simulink model "W6_cs"  (Simulink 8.3)
settings: Solver=ode4  SolverMode=SingleTasking  StartTime=0.0  StopTime=inf  FixedStep=1/60  RelTol=1e-3
model workspace (MAT data in the model file):
  mbox_table : struct (value not decoded)
  model_closed = 0
  sim_status = 0
PreLoadFcn:
  | check_NUTS_defined;
  | 
  | assignin('base',['model_closed_' bdroot],false);
InitFcn:
  | PreScanExperimentInitFcn(bdroot)
StopFcn:
  | PreScanExperimentStopFcn(bdroot)
  | close all;
  | 
  | format shortg
  | c = clock;
  | log_filename = ['log_EXT_',num2str(c(1)),'_',num2str(c(2)),'_',num2str(c(3)),'_',num2str(c(4)),'_',num2str(c(5)),'_',num2str(round(c(6)))];
  | save(log_filename,'res')
undefined symbols (not defined in the file): DiscIntNeverNeededParam, gray, warningInitialVelocity, x0
libraries: simulink x39, PreScanSimulinkLibrary x19, PreScanUsefulBlocks x10, simulink_extras x3, visionsources x2, dspsigops x2, dspnetwork x1, vrlib x1, visionsinks x1
(part 1 of 6)
CloseFcn:
  | evalin('base',['clear model_closed_' bdroot]);
settings Model: Creator=PRESCAN  LastModifiedBy=DrivingSim
settings DataIOCC: LimitDataPoints=off  SaveOutput=off  SignalLogging=off  DSMLogging=off  SaveTime=off
settings OptimizationCC: ExpressionDepthLimit=2147483647  InitFltsAndDblsToZero=on
settings DebuggingCC: SaveWithParameterizedLinksMsg=none  SignalResolutionControl=TryResolveAllWithWarning  SolverPrmCheckMsg=none  MultiTaskDSMMsg=warning  MultiTaskCondExecSysMsg=none  FcnCallInpInsideContextMsg=UseLocalSettings  FrameProcessingCompatibilityMsg=error
settings SFSimCC: SFSimEnableDebug=off  SFSimOverflowDetection=off  SFSimEcho=off
settings GRTTargetCC: TargetFcnLib=ansi_tfl_tmw.mat
settings ConfigComp: CovMetricSettings=dw  CovHtmlReporting=on  CovSaveCumulativeToWorkspaceVar=on  CovSaveSingleToWorkspaceVar=on  CovModelRefEnable=Off  CovExternalEMLEnable=off

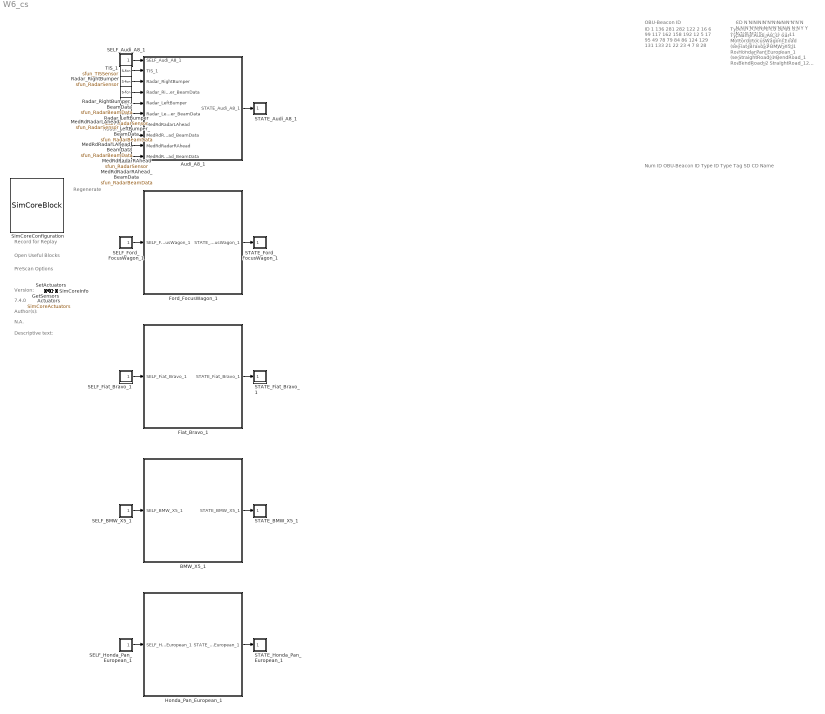
== system W6_cs ==
  note: Regenerate
  note: Record for Replay
  note: Open Useful Blocks
  note: PreScan Options
  note: Version:
  note: 7.4.0
  note: Author(s):
  note: N.A.
  note: Descriptive text:
  note: Num ID OBU-Beacon ID Type ID Type Tag SD CD Name
  note: ID
      |
      | 1
      | 136
      | 281
      | 282
      | 122
      | 2
      | 16
      | 6
      | 99
      | 117
      | 162
      | 158
      | 192
      | 12
      | 5
      | 17
      | 95
      | 49
      | 78
      | 79
      | 84
      | 86
      | 124
      | 129
      | 131
      | 133
      | 21
      | 22
      | 23
      | 4
      | 7
      | 8
      | 28
  note: OBU-Beacon ID
  note: TypeID
      |
      | 1
      | 1
      | 1
      | 1
      | 2
      | 11
      | 11
      | 11
      | 11
      | 11
      | 11
      | 11
      | 11
      | 11
      | 11
      | 11
      | 11
      | 11
      | 11
      | 11
      | 11
      | 11
      | 11
      | 11
      | 11
      | 11
      | 11
      | 11
      | 11
      | 11
      | 11
      | 11
      | 11
  note: TypeTag
      |
      | Car
      | Car
      | Car
      | Car
      | Motor
      | Road (segment)
      | Road (segment)
      | Road (segment)
      | Road (segment)
      | Road (segment)
      | Road (segment)
      | Road (segment)
      | Road (segment)
      | Road (segment)
      | Road (segment)
      | Road (segment)
      | Road (segment)
      | Road (segment)
      | Road (segment)
      | Road (segment)
      | Road (segment)
      | Road (segment)
      | Road (segment)
      | Road (segment)
      | Road (segment)
      | Road (segment)
      | Road (segment)
      | Road (segment)
      | Road (segment)
      | Road (segment)
      | Road (segment)
      | Road (segment)
      | Road (segment)
  note: SD
      |
      | Y
      | Y
      | N
      | N
      | N
      | Y
      | Y
      | Y
      | Y
      | Y
      | Y
      | Y
      | Y
      | Y
      | Y
      | Y
      | Y
      | Y
      | Y
      | Y
      | Y
      | Y
      | Y
      | Y
      | Y
      | Y
      | Y
      | Y
      | Y
      | Y
      | Y
      | Y
      | Y
  note: CD
      |
      | N
      | N
      | N
      | N
      | N
      | N
      | N
      | N
      | N
      | N
      | N
      | N
      | N
      | N
      | N
      | N
      | N
      | N
      | N
      | N
      | N
      | N
      | N
      | N
      | N
      | N
      | N
      | N
      | N
      | N
      | N
      | N
      | N
  note: Name
      |
      | Audi_A8_1
      | Ford_FocusWagon_1
      | Fiat_Bravo_1
      | BMW_X5_1
      | Honda_Pan_European_1
      | StraightRoad_1
      | BendRoad_1
      | BendRoad_2
      | StraightRoad_12
      | StraightRoad_20
      | BendRoad_19
      | BendRoad_17
      | StraightRoad_30
      | BendRoad_3
      | StraightRoad_2
      | BendRoad_4
      | StraightRoad_7
      | Ramp_3
      | Ramp_6
      | Ramp_7
      | Ramp_8
      | StraightRoad_8
      | StraightRoad_14
      | StraightRoad_15
      | BendRoad_11
      | StraightRoad_17
      | StraightRoad_13
      | StraightRoad_16
      | StraightRoad_9
      | StraightRoad_5
      | StraightRoad_3
      | StraightRoad_4
      | StraightRoad_6
  Actuators : DataStoreMemory  Tag=Actuators  DataStoreName=SimCoreActuators  InitialValue=zeros(75,1)
      settings: DeleteFcn=PreScanBlockDeleteFcn;
  Audi_A8_1 : Subsystem  Tag=WorldObjectSubSystem  InitFcn=|
      | UniqueId = '3687';
      | UniqueId = '4148';
      mask Display: image(imread('Audi_A8.jpg'));color('white');text(0,0,' ID=1\n')
  BMW_X5_1 : Subsystem  Tag=WorldObjectSubSystem  InitFcn=UniqueId = '5788';
      mask Display: image(imread('BMW_X5.jpg'));color('white');text(0,0,' ID=282\n')
  Fiat_Bravo_1 : Subsystem  Tag=WorldObjectSubSystem  InitFcn=UniqueId = '4829';
      mask Display: image(imread('Fiat_Bravo.jpg'));color('white');text(0,0,' ID=281\n')
  Ford_FocusWagon_1 : Subsystem  Tag=WorldObjectSubSystem  InitFcn=UniqueId = '4410';
      mask Display: image(imread('Ford_FocusWagon.jpg'));color('white');text(0,0,' ID=136\n')
  GetSensors : Subsystem  Tag=GetSensors  Priority=2  mask(PreScan Simulation Core Block){NrOfSensors=40, TimeStep=1/60}
      mask prompts: NrOfSensors "Number of sensor values"; TimeStep "Timestep [s]"
      mask help:
      | Please do not remove this block from the PreScan compilation sheet,
      | as it contains essential configuration parameters for a PreScan simulation.
      settings: DeleteFcn=PreScanBlockDeleteFcn;
  Honda_Pan_European_1 : Subsystem  Tag=WorldObjectSubSystem  InitFcn=UniqueId = '6490';
      mask Display: image(imread('Honda_Pan_European.jpg'));color('white');text(0,0,' ID=122\n')
  MedRdRadarLAhead : S-Function  Priority=3  LoadFcn=load('PrescanScannerSensorData.mat');load('PrescanScannerSensorMessage.mat')  FunctionName=sfun_RadarSensor  Parameters=timestepMask maxInputMessages maxOutputMessages sensorID detectableObjects  EnableBusSupport=off  mask{timestepMask=1/60, maxInputMessages=0, maxOutputMessages=1, sensorID=6836, detectableObjects=1}
      mask prompts: timestepMask "MATLAB timestep:"; maxInputMessages "Max input messages:"; maxOutputMessages "Max output messages:"; sensorID "Sensor ID:"; detectableObjects "Max detectable objects:"
      mask help: RadarSensor I/O
      mask Display: image(imread('Radar.png'))
  MedRdRadarLAhead_BeamData : S-Function  Priority=3  LoadFcn=load('PrescanScannerSensorBeamData.mat');load('PrescanScannerSensorBeamMessage.mat')  FunctionName=sfun_RadarBeamData  Parameters=timestepMask maxInputMessages maxOutputMessages sensorID detectableObjects  EnableBusSupport=off  mask{timestepMask=1/60, maxInputMessages=0, maxOutputMessages=1, sensorID=6836, detectableObjects=1}
      mask prompts: timestepMask "MATLAB timestep:"; maxInputMessages "Max input messages:"; maxOutputMessages "Max output messages:"; sensorID "Sensor ID:"; detectableObjects "Max detectable objects:"
      mask help: RadarSensor I/O
      mask Display: image(imread('BeamInfo.png'))
  MedRdRadarRAhead : S-Function  Priority=3  LoadFcn=load('PrescanScannerSensorData.mat');load('PrescanScannerSensorMessage.mat')  FunctionName=sfun_RadarSensor  Parameters=timestepMask maxInputMessages maxOutputMessages sensorID detectableObjects  EnableBusSupport=off  mask{timestepMask=1/60, maxInputMessages=0, maxOutputMessages=1, sensorID=6837, detectableObjects=1}
      mask prompts: timestepMask "MATLAB timestep:"; maxInputMessages "Max input messages:"; maxOutputMessages "Max output messages:"; sensorID "Sensor ID:"; detectableObjects "Max detectable objects:"
      mask help: RadarSensor I/O
      mask Display: image(imread('Radar.png'))
  MedRdRadarRAhead_BeamData : S-Function  Priority=3  LoadFcn=load('PrescanScannerSensorBeamData.mat');load('PrescanScannerSensorBeamMessage.mat')  FunctionName=sfun_RadarBeamData  Parameters=timestepMask maxInputMessages maxOutputMessages sensorID detectableObjects  EnableBusSupport=off  mask{timestepMask=1/60, maxInputMessages=0, maxOutputMessages=1, sensorID=6837, detectableObjects=1}
      mask prompts: timestepMask "MATLAB timestep:"; maxInputMessages "Max input messages:"; maxOutputMessages "Max output messages:"; sensorID "Sensor ID:"; detectableObjects "Max detectable objects:"
      mask help: RadarSensor I/O
      mask Display: image(imread('BeamInfo.png'))
  Radar_LeftBumper : S-Function  Priority=3  LoadFcn=load('PrescanScannerSensorData.mat');load('PrescanScannerSensorMessage.mat')  FunctionName=sfun_RadarSensor  Parameters=timestepMask maxInputMessages maxOutputMessages sensorID detectableObjects  EnableBusSupport=off  mask{timestepMask=1/60, maxInputMessages=0, maxOutputMessages=1, sensorID=6637, detectableObjects=1}
      mask prompts: timestepMask "MATLAB timestep:"; maxInputMessages "Max input messages:"; maxOutputMessages "Max output messages:"; sensorID "Sensor ID:"; detectableObjects "Max detectable objects:"
      mask help: RadarSensor I/O
      mask Display: image(imread('Radar.png'))
  Radar_LeftBumper_BeamData : S-Function  Priority=3  LoadFcn=load('PrescanScannerSensorBeamData.mat');load('PrescanScannerSensorBeamMessage.mat')  FunctionName=sfun_RadarBeamData  Parameters=timestepMask maxInputMessages maxOutputMessages sensorID detectableObjects  EnableBusSupport=off  mask{timestepMask=1/60, maxInputMessages=0, maxOutputMessages=1, sensorID=6637, detectableObjects=1}
      mask prompts: timestepMask "MATLAB timestep:"; maxInputMessages "Max input messages:"; maxOutputMessages "Max output messages:"; sensorID "Sensor ID:"; detectableObjects "Max detectable objects:"
      mask help: RadarSensor I/O
      mask Display: image(imread('BeamInfo.png'))
  Radar_RightBumper : S-Function  Priority=3  LoadFcn=load('PrescanScannerSensorData.mat');load('PrescanScannerSensorMessage.mat')  FunctionName=sfun_RadarSensor  Parameters=timestepMask maxInputMessages maxOutputMessages sensorID detectableObjects  EnableBusSupport=off  mask{timestepMask=1/60, maxInputMessages=0, maxOutputMessages=1, sensorID=6636, detectableObjects=1}
      mask prompts: timestepMask "MATLAB timestep:"; maxInputMessages "Max input messages:"; maxOutputMessages "Max output messages:"; sensorID "Sensor ID:"; detectableObjects "Max detectable objects:"
      mask help: RadarSensor I/O
      mask Display: image(imread('Radar.png'))
  Radar_RightBumper_BeamData : S-Function  Priority=3  LoadFcn=load('PrescanScannerSensorBeamData.mat');load('PrescanScannerSensorBeamMessage.mat')  FunctionName=sfun_RadarBeamData  Parameters=timestepMask maxInputMessages maxOutputMessages sensorID detectableObjects  EnableBusSupport=off  mask{timestepMask=1/60, maxInputMessages=0, maxOutputMessages=1, sensorID=6636, detectableObjects=1}
      mask prompts: timestepMask "MATLAB timestep:"; maxInputMessages "Max input messages:"; maxOutputMessages "Max output messages:"; sensorID "Sensor ID:"; detectableObjects "Max detectable objects:"
      mask help: RadarSensor I/O
      mask Display: image(imread('BeamInfo.png'))
  SELF_Audi_A8_1 : Subsystem  Tag=SELF  Priority=3  mask(PreScan Source Block: SELF){PortName=SELF_Audi_A8_1, PortIndex=0, PortWidth=8, TimeStep=1/60}
      mask prompts: PortName "Auto-Assigned: Port Name [-]"; PortIndex "Auto-Assigned: Port Index [-]"; PortWidth "Auto-Assigned: Port Dimensions"; TimeStep "Auto-Assigned: Upload Period [s]"
      mask help:
      | The SELF port shows (state) information of the actor itself. The outputs are position in the experiment's axis system and the GPS coordinates, and the object's absolute velocity and compass heading.
      |
      | For more information, please click Help.
      settings: DeleteFcn=PreScanBlockDeleteFcn;
      mask Help: eval('openHelp(462)')
      mask Display: image(imread('GPS.png'))
  SELF_BMW_X5_1 : Subsystem  Tag=SELF  Priority=3  mask(PreScan Source Block: SELF){PortName=SELF_BMW_X5_1, PortIndex=24, PortWidth=8, TimeStep=1/60}
      mask prompts: PortName "Auto-Assigned: Port Name [-]"; PortIndex "Auto-Assigned: Port Index [-]"; PortWidth "Auto-Assigned: Port Dimensions"; TimeStep "Auto-Assigned: Upload Period [s]"
      mask help:
      | The SELF port shows (state) information of the actor itself. The outputs are position in the experiment's axis system and the GPS coordinates, and the object's absolute velocity and compass heading.
      |
      | For more information, please click Help.
      settings: DeleteFcn=PreScanBlockDeleteFcn;
      mask Help: eval('openHelp(462)')
      mask Display: image(imread('GPS.png'))
  SELF_Fiat_Bravo_1 : Subsystem  Tag=SELF  Priority=3  mask(PreScan Source Block: SELF){PortName=SELF_Fiat_Bravo_1, PortIndex=16, PortWidth=8, TimeStep=1/60}
      mask prompts: PortName "Auto-Assigned: Port Name [-]"; PortIndex "Auto-Assigned: Port Index [-]"; PortWidth "Auto-Assigned: Port Dimensions"; TimeStep "Auto-Assigned: Upload Period [s]"
      mask help:
      | The SELF port shows (state) information of the actor itself. The outputs are position in the experiment's axis system and the GPS coordinates, and the object's absolute velocity and compass heading.
      |
      | For more information, please click Help.
      settings: DeleteFcn=PreScanBlockDeleteFcn;
      mask Help: eval('openHelp(462)')
      mask Display: image(imread('GPS.png'))
  SELF_Ford_FocusWagon_1 : Subsystem  Tag=SELF  Priority=3  mask(PreScan Source Block: SELF){PortName=SELF_Ford_FocusWagon_1, PortIndex=8, PortWidth=8, TimeStep=1/60}
      mask prompts: PortName "Auto-Assigned: Port Name [-]"; PortIndex "Auto-Assigned: Port Index [-]"; PortWidth "Auto-Assigned: Port Dimensions"; TimeStep "Auto-Assigned: Upload Period [s]"
      mask help:
      | The SELF port shows (state) information of the actor itself. The outputs are position in the experiment's axis system and the GPS coordinates, and the object's absolute velocity and compass heading.
      |
      | For more information, please click Help.
      settings: DeleteFcn=PreScanBlockDeleteFcn;
      mask Help: eval('openHelp(462)')
      mask Display: image(imread('GPS.png'))
  SELF_Honda_Pan_European_1 : Subsystem  Tag=SELF  Priority=3  mask(PreScan Source Block: SELF){PortName=SELF_Honda_Pan_European_1, PortIndex=32, PortWidth=8, TimeStep=1/60}
      mask prompts: PortName "Auto-Assigned: Port Name [-]"; PortIndex "Auto-Assigned: Port Index [-]"; PortWidth "Auto-Assigned: Port Dimensions"; TimeStep "Auto-Assigned: Upload Period [s]"
      mask help:
      | The SELF port shows (state) information of the actor itself. The outputs are position in the experiment's axis system and the GPS coordinates, and the object's absolute velocity and compass heading.
      |
      | For more information, please click Help.
      settings: DeleteFcn=PreScanBlockDeleteFcn;
      mask Help: eval('openHelp(462)')
      mask Display: image(imread('GPS.png'))
  STATE_Audi_A8_1 : Subsystem  Tag=State  Priority=0  mask(PreScan Sink Block: State){x0=-399.91707801225488, y0=254.16247682781102, z0=0.55, Roll0=0, Pitch0=0, Yaw0=339.99999999999989, TimeStep=1/60}
      mask prompts: x0 "Ini x-position VEHICLE wrt GLOBAL axis system [m]"; y0 "Ini y-position VEHICLE wrt GLOBAL axis system [m]"; z0 "Ini z-position VEHICLE wrt GLOBAL axis system [m]"; Roll0 "Ini roll-angle BODY wrt VEHICLE axis system [deg]"; Pitch0 "Ini pitch-angle BODY wrt VEHICLE axis system [deg]"; Yaw0 "Ini yaw-angle VEHICLE wrt GLOBAL axis system [deg]"; TimeStep "Time Step [s]"
      mask help:
      | The Actor State contains a vector signal of size (9x1), containing the following signals:
      |
      | -  Position                  (x,y,z)                                     [m]
      | -  Velocity                  (vx,vy,vz)                               [m/s]
      | -  Angles                    (Roll, Pitch, Yaw)                   [rad]
      |
      | The Actor state is defined in the global axis system.
      | The state is superponed on the Initial position defined in the GUI.
      |
      | For more information, please click Help.
      settings: DeleteFcn=PreScanBlockDeleteFcn;
      mask Help: eval('openHelp(222)')
      mask Display: image(imread('State.png'))
  STATE_BMW_X5_1 : Subsystem  Tag=State  Priority=0  mask(PreScan Sink Block: State){x0=-66.9525002880753, y0=135.98733029367131, z0=0.69, Roll0=0, Pitch0=0, Yaw0=160.19495482924066, TimeStep=1/60}
      mask prompts: x0 "Ini x-position VEHICLE wrt GLOBAL axis system [m]"; y0 "Ini y-position VEHICLE wrt GLOBAL axis system [m]"; z0 "Ini z-position VEHICLE wrt GLOBAL axis system [m]"; Roll0 "Ini roll-angle BODY wrt VEHICLE axis system [deg]"; Pitch0 "Ini pitch-angle BODY wrt VEHICLE axis system [deg]"; Yaw0 "Ini yaw-angle VEHICLE wrt GLOBAL axis system [deg]"; TimeStep "Time Step [s]"
      mask help:
      | The Actor State contains a vector signal of size (9x1), containing the following signals:
      |
      | -  Position                  (x,y,z)                                     [m]
      | -  Velocity                  (vx,vy,vz)                               [m/s]
      | -  Angles                    (Roll, Pitch, Yaw)                   [rad]
      |
      | The Actor state is defined in the global axis system.
      | The state is superponed on the Initial position defined in the GUI.
      |
      | For more information, please click Help.
      settings: DeleteFcn=PreScanBlockDeleteFcn;
      mask Help: eval('openHelp(222)')
      mask Display: image(imread('State.png'))
  STATE_Fiat_Bravo_1 : Subsystem  Tag=State  Priority=0  mask(PreScan Sink Block: State){x0=870.78469646749215, y0=-350.59511540043718, z0=0.56, Roll0=0, Pitch0=0, Yaw0=72.606570567857887, TimeStep=1/60}
      mask prompts: x0 "Ini x-position VEHICLE wrt GLOBAL axis system [m]"; y0 "Ini y-position VEHICLE wrt GLOBAL axis system [m]"; z0 "Ini z-position VEHICLE wrt GLOBAL axis system [m]"; Roll0 "Ini roll-angle BODY wrt VEHICLE axis system [deg]"; Pitch0 "Ini pitch-angle BODY wrt VEHICLE axis system [deg]"; Yaw0 "Ini yaw-angle VEHICLE wrt GLOBAL axis system [deg]"; TimeStep "Time Step [s]"
      mask help:
      | The Actor State contains a vector signal of size (9x1), containing the following signals:
      |
      | -  Position                  (x,y,z)                                     [m]
      | -  Velocity                  (vx,vy,vz)                               [m/s]
      | -  Angles                    (Roll, Pitch, Yaw)                   [rad]
      |
      | The Actor state is defined in the global axis system.
      | The state is superponed on the Initial position defined in the GUI.
      |
      | For more information, please click Help.
      settings: DeleteFcn=PreScanBlockDeleteFcn;
      mask Help: eval('openHelp(222)')
      mask Display: image(imread('State.png'))
  STATE_Ford_FocusWagon_1 : Subsystem  Tag=State  Priority=0  mask(PreScan Sink Block: State){x0=-113.09931945800781, y0=149.31063842773437, z0=0.5, Roll0=0, Pitch0=0, Yaw0=340.09422131164354, TimeStep=1/60}
      mask prompts: x0 "Ini x-position VEHICLE wrt GLOBAL axis system [m]"; y0 "Ini y-position VEHICLE wrt GLOBAL axis system [m]"; z0 "Ini z-position VEHICLE wrt GLOBAL axis system [m]"; Roll0 "Ini roll-angle BODY wrt VEHICLE axis system [deg]"; Pitch0 "Ini pitch-angle BODY wrt VEHICLE axis system [deg]"; Yaw0 "Ini yaw-angle VEHICLE wrt GLOBAL axis system [deg]"; TimeStep "Time Step [s]"
      mask help:
      | The Actor State contains a vector signal of size (9x1), containing the following signals:
      |
      | -  Position                  (x,y,z)                                     [m]
      | -  Velocity                  (vx,vy,vz)                               [m/s]
      | -  Angles                    (Roll, Pitch, Yaw)                   [rad]
      |
      | The Actor state is defined in the global axis system.
      | The state is superponed on the Initial position defined in the GUI.
      |
      | For more information, please click Help.
      settings: DeleteFcn=PreScanBlockDeleteFcn;
      mask Help: eval('openHelp(222)')
      mask Display: image(imread('State.png'))
  STATE_Honda_Pan_European_1 : Subsystem  Tag=State  Priority=0  mask(PreScan Sink Block: State){x0=1149.497802734375, y0=222.82337188720703, z0=0.5949, Roll0=0, Pitch0=0, Yaw0=170, TimeStep=1/60}
      mask prompts: x0 "Ini x-position VEHICLE wrt GLOBAL axis system [m]"; y0 "Ini y-position VEHICLE wrt GLOBAL axis system [m]"; z0 "Ini z-position VEHICLE wrt GLOBAL axis system [m]"; Roll0 "Ini roll-angle BODY wrt VEHICLE axis system [deg]"; Pitch0 "Ini pitch-angle BODY wrt VEHICLE axis system [deg]"; Yaw0 "Ini yaw-angle VEHICLE wrt GLOBAL axis system [deg]"; TimeStep "Time Step [s]"
      mask help:
      | The Actor State contains a vector signal of size (9x1), containing the following signals:
      |
      | -  Position                  (x,y,z)                                     [m]
      | -  Velocity                  (vx,vy,vz)                               [m/s]
      | -  Angles                    (Roll, Pitch, Yaw)                   [rad]
      |
      | The Actor state is defined in the global axis system.
      | The state is superponed on the Initial position defined in the GUI.
      |
      | For more information, please click Help.
      settings: DeleteFcn=PreScanBlockDeleteFcn;
      mask Help: eval('openHelp(222)')
      mask Display: image(imread('State.png'))
  SetActuators : Subsystem  Tag=SetActuators  Priority=1  mask(PreScan Simulation Core Block){TimeStep=1/60, NrOfActuators=75}
      mask prompts: TimeStep "Timestep [s]"; NrOfActuators "Number of actuator values"
      mask help:
      | Please do not remove this block from the PreScan compilation sheet,
      | as it contains essential configuration parameters for a PreScan simulation.
      settings: DeleteFcn=PreScanBlockDeleteFcn;
  SimCoreConfiguration : M-S-Function  Tag=SimCoreConfiguration  Description=2DB88F1AB85D6AB0C7A46FBF0985E444AD6743D233D065952F88CD829B0DCDCE  FunctionName=SimCoreBlock  Parameters=ExperimentXML PortsXML SimulationCore HostName CheckStart EnableLog RfR EnableGPUAccel ShowComputationTime  mask(PreScan Simulation Core Configurator){SimulationCore=NUTS, HostName=0, CheckStart=0, prescanversion='7.4.0', EnableLog=off, RfR=0, EnableGPUAccel=on, ShowComputationTime=off}
      mask prompts: SimulationCore "Simulation Core"; HostName "Simulation Host"; CheckStart "Show START Dialog"; prescanversion "PreScan Version"; EnableLog "Create TA Log"; RfR "Record for Replay"; EnableGPUAccel "Enable GPU Acceleration"; ShowComputationTime "Show ComputationTime Scope"
      mask help:
      | Please do not remove this block from the PreScan compilation sheet,
      | as it contains essential configuration parameter for a PreScan simulation.
      mask init:
      | model = bdroot;
      | ExperimentXML = [model(1:end-3) '.pex'];
      | PortsXML = [model '_ports.pcd'];
      settings: DeleteFcn=PreScanBlockDeleteFcn;  ModelCloseFcn=assignin('base',['model_closed_' bdroot],true);
      mask Help: eval('openHelp(812)')
      mask Display: image(imread('prescanlogo.ico'))
  SimCoreInfo : Subsystem  Tag=SimCoreInfo
  TIS_1 : S-Function  Priority=3  LoadFcn=load('PrescanScannerSensorData.mat');load('PrescanScannerSensorMessage.mat')  FunctionName=sfun_TISSensor  Parameters=timestepMask maxInputMessages maxOutputMessages sensorID detectableObjects  EnableBusSupport=off  mask{timestepMask=1/60, maxInputMessages=0, maxOutputMessages=1, sensorID=4973, detectableObjects=1}
      mask prompts: timestepMask "MATLAB timestep:"; maxInputMessages "Max input messages:"; maxOutputMessages "Max output messages:"; sensorID "Sensor ID:"; detectableObjects "Max detectable objects:"
      mask help: TIS Sensor I/O
      mask Display: image(imread('TIS.png'))
  wires:
  SetActuators/1(dummy) -> GetSensors/1(dummy)
  Audi_A8_1/1(STATE_Audi_A8_1) -> STATE_Audi_A8_1/1(State)
  SELF_Audi_A8_1/1(U) -> Audi_A8_1/1(SELF_Audi_A8_1)
  TIS_1/1 -> Audi_A8_1/2(TIS_1)
  Radar_RightBumper/1 -> Audi_A8_1/3(Radar_RightBumper)
  Radar_RightBumper_BeamData/1 -> Audi_A8_1/4(Radar_RightBumper_BeamData)
  Radar_LeftBumper/1 -> Audi_A8_1/5(Radar_LeftBumper)
  Radar_LeftBumper_BeamData/1 -> Audi_A8_1/6(Radar_LeftBumper_BeamData)
  MedRdRadarLAhead/1 -> Audi_A8_1/7(MedRdRadarLAhead)
  MedRdRadarLAhead_BeamData/1 -> Audi_A8_1/8(MedRdRadarLAhead_BeamData)
  MedRdRadarRAhead/1 -> Audi_A8_1/9(MedRdRadarRAhead)
  MedRdRadarRAhead_BeamData/1 -> Audi_A8_1/10(MedRdRadarRAhead_BeamData)
  Ford_FocusWagon_1/1(STATE_Ford_FocusWagon_1) -> STATE_Ford_FocusWagon_1/1(State)
  SELF_Ford_FocusWagon_1/1(U) -> Ford_FocusWagon_1/1(SELF_Ford_FocusWagon_1)
  Fiat_Bravo_1/1(STATE_Fiat_Bravo_1) -> STATE_Fiat_Bravo_1/1(State)
  SELF_Fiat_Bravo_1/1(U) -> Fiat_Bravo_1/1(SELF_Fiat_Bravo_1)
  BMW_X5_1/1(STATE_BMW_X5_1) -> STATE_BMW_X5_1/1(State)
  SELF_BMW_X5_1/1(U) -> BMW_X5_1/1(SELF_BMW_X5_1)
  Honda_Pan_European_1/1(STATE_Honda_Pan_European_1) -> STATE_Honda_Pan_European_1/1(State)
  SELF_Honda_Pan_European_1/1(U) -> Honda_Pan_European_1/1(SELF_Honda_Pan_European_1)

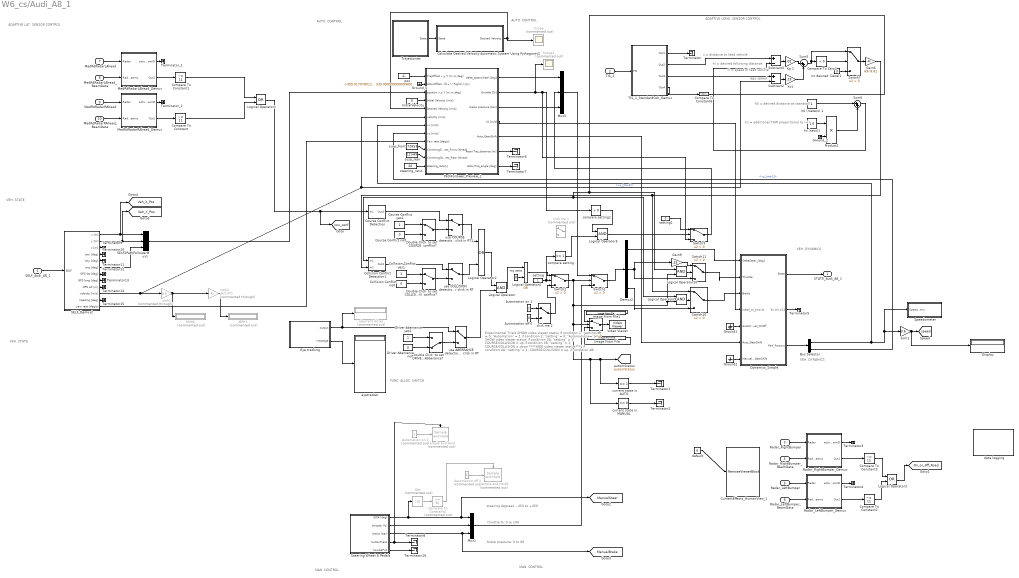
== system W6_cs/Audi_A8_1 ==
  note: Experimental Trials
      | SHOW video viewer status
      | if condition 1; ''setting'' = 0; ''Automation'' = 1
      | if condition 2; ''setting'' = 0; ''Automation'' = 1
      |
      | SHOW video viewer status
      | if condition 3A; ''setting'' = 1; COURSE/COLLISION = up
      | if condition 3B; ''setting'' = 1; COURSE/COLLISION = down
      |
      | ****HIDE video viewer status****
      | if condition 4A; ''setting'' = 1; COURSE/COLLISION = up,
      | if condition 4B; ''setting'' = 1; COURSE/COLLISION = down
      | if condition 4C; "setting"= 0; "Automation" = 0
  note: hi = desired following distance
  note: x = distance to lead vehicle
  note: vi = speed of lead vehicle
  note: hv = additional THW proportional to (vi)
  note: h0 = desired distance at standstill
  note: VEH. STATE
  note: VEH. STATE
  note: AUTO. CONTROL
  note: AUTO. CONTROL
  note: VEH. DYNAMICS
  note: VEH. DYNAMICS
  note: FUNC. ALLOC. SWITCH
  note: throttle %: 0 to 100
  note: brake pressure: 0 to 69
  note: steering degrees: - 450 to +450
  note: MAN. CONTROL
  note: MAN. CONTROL
  note: ADAPTIVE LONG. SENSOR CONTROL
  note: ADAPTIVE LAT. SENSOR CONTROL
  note: ego speed
  SELF_Audi_A8_1 : Inport  Tag=SELFInport
  TIS_1 : Inport  Tag=RadarInport  Port=2  OutDataTypeStr=Bus: PRESCAN_SCANNERSENSORMESSAGE
  Radar_RightBumper : Inport  Tag=RadarInport  Port=3  OutDataTypeStr=Bus: PRESCAN_SCANNERSENSORMESSAGE
  Radar_RightBumper_BeamData : Inport  Tag=RadarInport  Port=4  OutDataTypeStr=Bus: PRESCAN_SCANNERSENSORBEAMMESSAGE
  Radar_LeftBumper : Inport  Tag=RadarInport  Port=5  OutDataTypeStr=Bus: PRESCAN_SCANNERSENSORMESSAGE
  Radar_LeftBumper_BeamData : Inport  Tag=RadarInport  Port=6  OutDataTypeStr=Bus: PRESCAN_SCANNERSENSORBEAMMESSAGE
  MedRdRadarLAhead : Inport  Tag=RadarInport  Port=7  OutDataTypeStr=Bus: PRESCAN_SCANNERSENSORMESSAGE
  MedRdRadarLAhead_BeamData : Inport  Tag=RadarInport  Port=8  OutDataTypeStr=Bus: PRESCAN_SCANNERSENSORBEAMMESSAGE
  MedRdRadarRAhead : Inport  Tag=RadarInport  Port=9  OutDataTypeStr=Bus: PRESCAN_SCANNERSENSORMESSAGE
  MedRdRadarRAhead_BeamData : Inport  Tag=RadarInport  Port=10  OutDataTypeStr=Bus: PRESCAN_SCANNERSENSORBEAMMESSAGE
  Abs : Abs  Commented=on
  Autiomation off 0 : Constant  Value=0
  Automation off 3 : Constant  Commented=on  Value=0
  Automation on 1 : Constant
  Automation on 2 : Constant  Commented=on
  Bus Selector : BusSelector  OutputSignals=vx_[ms-1],vy_[ms-1]
  Calculate Desired Velocity Automatic System Using Pythagoras2 : Subsystem
  Collision Conflict Detection1 : Subsystem
  Collision Conflict no0 : Constant  Value=0
  Collision Conflict yes1 : Constant
  Compare To Constant{,1..3} (4 alike) : simulink/Logic and Bit Operations/Compare To Constant  relop=~=  const=11  OutDataTypeStr=boolean
  Compare To Constant4 : simulink/Logic and Bit Operations/Compare To Constant  Commented=on  relop=>=  const=90  OutDataTypeStr=boolean
  Compare To Constant6 : simulink/Logic and Bit Operations/Compare To Constant  relop===  const=1  OutDataTypeStr=boolean
  Compare To Zero1 : simulink/Logic and Bit Operations/Compare To Zero  relop=<  OutDataTypeStr=boolean
  Course Conflict Detection : Subsystem
  Course Conflict no0 : Constant  Value=0
  Course Conflict yes1 : Constant
  CurrentEffects_HumanView_1 : M-S-Function  FunctionName=RemoteViewerBlock  Parameters=2
  Demux2 : Demux  Outputs=3
  Display : Display
  Double Click  to set COLLISION  conflict? : ManualSwitch
  Double Click  to set COURSE  conflict? : ManualSwitch
  Double Click  to set DRIVER  Abberance? : ManualSwitch  CurrentSetting=0
  Driver Aberrance no0 : Constant  Value=0
  Driver Aberrance yes1 : Constant
  Dynamics_Simple : Subsystem  Tag=Simple_Vehicle_Dynamics  mask(PreScan Block: Simple Dynamics){Migrate=on, TimeStep=1/60, ComputationMode=Continuous_Time}
      mask prompts: Migrate "Migrate. During migration this block will be replaced by a newer one."; TimeStep "Auto assigned: Time Step [s]"; ComputationMode "Computation mode:"
      mask help:
      | The Simple Dynamics Model is selected in the GUI to simulate vehicle dynamics behavior.
      |
      | The Simple Dynamics Model is completely open to the user. The parameters of this model can be set in the Simple Dynamics dialog in the GUI.
      |
      | For more information, please click Help.
      mask init:
      | p = SimpleDyn_pars;
      settings: DeleteFcn=PreScanBlockDeleteFcn;
      mask Help: eval('openHelp(220)')
      mask Display:
      | image(imread('SimpleDyn.png'))
      | port_label('input', 1, '{\delta}_S_t_ _e_e_r [deg]','texmode','on')
      | port_label('input', 2, 'Throttle [%]')
      | port_label('input', 3, 'Brake Pres [bar]')
      | port_label('input', 4, 'V_0 [ms-1]','texmode','on')
      | port_label('input', 5, 'Auto=[0]/Manual=[1]')
      | port_label('input', 6, 'Auto_GearShift')
      | port_label('input', 7, 'Manual_GearShift')
      | port_label('output', 1, 'State')
      | port_label('output', 2, 'Vx [ms-1]')
      | port_label('output', 3, 'Perf Params')
  Eye tracking : Subsystem
  Gain6 : Gain  Gain=69/-9.81
  Gain9 : Gain  Gain=.25
  Ground1 : Ground
  Ground2 : Ground
  Ground_1 : Ground
  Ground_2 : Ground
  Image From File : visionsources/Image From File  Tag=vipblks_nd  FileName=NormalDrivingGreen.png  imagePorts=One multidimensional signal  Ts=inf  ImageDataType=Inherit from input image  Signed=on  WordLength=16  sdImageDataType=uint(8)  FractionLengthMode=User-defined  FractionLength=15  OutPortLabels=R|G|B
  Image From File1 : visionsources/Image From File  Tag=vipblks_nd  FileName=AutoBackupControlRed.png  imagePorts=One multidimensional signal  Ts=inf  ImageDataType=Inherit from input image  Signed=on  WordLength=16  sdImageDataType=uint(8)  FractionLengthMode=User-defined  FractionLength=15  OutPortLabels=R|G|B
  InitialVelocity : Constant  Tag=InitialVelocity  Value=0
  KMH1 : Display  Commented=on
  Kp 1 : Gain  Gain=.02
  Kv1 : Gain  Gain=.23
  Logical Operator{,5,9..10} (4 alike) : Logic  AllPortsSameDT=off  OutDataTypeStr=boolean
  Logical Operator{1..4} (4 alike) : Logic  Operator=OR  AllPortsSameDT=off  OutDataTypeStr=boolean
  MPH1 : Display  Commented=on
  MedRdRadarLAhead_Demux : Subsystem  TreatAsAtomicUnit=on  mask(PreScan Demux Block: Radar){MAXMESSAGES=1}
      mask prompts: MAXMESSAGES "Number of Objects"
      mask help:
      | The Radar Sensor is a detailed sensor based on a physical radar
      | model that includes Antenna GAIN Maps (AGM) and atmospheric
      | attenuation.
      |
      | For more information, please click Help.
      mask Help: eval('openHelp(431)')
      mask Display:
      | port_label('input',1,'Radar')
      | port_label('output',1,'Radar Data')
  MedRdRadarRAhead_Demux : Subsystem  TreatAsAtomicUnit=on  mask(PreScan Demux Block: Radar){MAXMESSAGES=1}
      mask prompts: MAXMESSAGES "Number of Objects"
      mask help:
      | The Radar Sensor is a detailed sensor based on a physical radar
      | model that includes Antenna GAIN Maps (AGM) and atmospheric
      | attenuation.
      |
      | For more information, please click Help.
      mask Help: eval('openHelp(431)')
      mask Display:
      | port_label('input',1,'Radar')
      | port_label('output',1,'Radar Data')
  Mux1 : Mux  Inputs=3
  Mux3 : Mux  Inputs=3
  PathFollower_Preview_1 : Subsystem  Tag=PathFollower_Preview  mask(PreScan Block: Path Follower with Preview){Migrate=on, FileName='Trajectory_1.mat', mass=1820, Jzz=3746, length_a=2.94 - 1.77, length_l=2.94, Angle_Max_SteeringWheel=500, PreviewTime=1, DelayTime=0.1, LowSpeedLimit=20, MaxSteeringRate=1200, CSSampleTime=1/60, PFIntegrationFrequency=60}
      mask prompts: Migrate "Migrate. During migration this block will be replaced by a newer one."; FileName "Trajectory Name"; mass "Mass vehicle total [kg]"; Jzz "Inertia vehicle around yaw axis [kg m2]"; length_a "Distance between COG and front axle [m]"; length_l "Length of wheelbase [m]"; Angle_Max_SteeringWheel "Maximum steering wheel angle [deg]"; PreviewTime "Preview time [s]"; DelayTime "Delay time [s]"; LowSpeedLimit "Low-speed limit [km/h]"; MaxSteeringRate "Maximum steering wheel angle rate [deg/s]"; CSSampleTime "Compilation Sheet sample time [s]"; PFIntegrationFrequency "Lateral controller frequency [Hz]"
      mask help:
      | The Path Follower Model is selected in the GUI to simulate driver behavior.
      |
      | For more information, please click Help.
      mask init:
      | load(['trajectories/',eval(FileName)])
      | traject=trajectory';
      | 
      | Traj_x=traject(:,2);
      | Traj_y=traject(:,3);
      | Traj_t=traject(2,1);
      | Traj_v=sqrt(traject(:,8).^2+traject(:,9).^2+traject(:,10).^2);
      | 
      | RefreshCounter = (1/CSSampleTime) / (PFIntegrationFrequency); %Compilation sheet frequency/path follower frequency
      | 
      | blockPath = gcb;
      | 
      | clear traject;
      mask Help: eval('openHelp(233)')
  Product1 : Product
  Radar_LeftBumper_Demux : Subsystem  TreatAsAtomicUnit=on  mask(PreScan Demux Block: Radar){MAXMESSAGES=1}
      mask prompts: MAXMESSAGES "Number of Objects"
      mask help:
      | The Radar Sensor is a detailed sensor based on a physical radar
      | model that includes Antenna GAIN Maps (AGM) and atmospheric
      | attenuation.
      |
      | For more information, please click Help.
      mask Help: eval('openHelp(431)')
      mask Display:
      | port_label('input',1,'Radar')
      | port_label('output',1,'Radar Data')
  Radar_RightBumper_Demux : Subsystem  TreatAsAtomicUnit=on  mask(PreScan Demux Block: Radar){MAXMESSAGES=1}
      mask prompts: MAXMESSAGES "Number of Objects"
      mask help:
      | The Radar Sensor is a detailed sensor based on a physical radar
      | model that includes Antenna GAIN Maps (AGM) and atmospheric
      | attenuation.
      |
      | For more information, please click Help.
      mask Help: eval('openHelp(431)')
      mask Display:
      | port_label('input',1,'Radar')
      | port_label('output',1,'Radar Data')
  SELF2PathFollowerMux1 : Mux  Inputs=3
  SELF_Demux2 : Subsystem  Tag=DemuxSELF  mask(PreScan Demux Block:){}
      settings: DeleteFcn=PreScanBlockDeleteFcn;
      mask Display:
      | port_label('output',1,'x [m]')
      | port_label('output',2,'y [m]')
      | port_label('output',3,'z [m]','texmode','on')
      | port_label('output',4,'Rotx [deg]','texmode','on')
      | port_label('output',5,'Roty [deg]','texmode','on')
      | port_label('output',6,'Rotz [deg]','texmode','on')
      | port_label('output',7,'GPS lat [deg]','texmode','on')
      | port_label('output',8,'GPS long [deg]','texmode','on')
      | port_label('output',9,'GPS alt [m]','texmode','on')
      | port_label('output',10,'Velocity [m/s]')
      | port_label('output',11,'Heading [deg]')
      | port_label('output',12,'Yaw rate [deg/s]')
  Sample and Hold : dspsigops/Sample and Hold  Commented=on  trig=Rising edge  initCond=0  latchinput=off
  Sample and Hold1 : dspsigops/Sample and Hold  Commented=on  trig=Rising edge  initCond=1  latchinput=off
  Scope : Scope  Commented=on
      settings: YMin=0  YMax=20
  Scope1 : Scope  Commented=on
      settings: YMin=0  YMax=20
  Speedometer : Subsystem
      mask init:
      | FigHandle = figure(101);
      | set(FigHandle, 'Position', [2150, -275, 400, 400]);
      | set(gcf,'Color','None');
      | ha = axes('units','normalized', 'position',[0,0,1,1]);
      | bg = imread('2016_Audi.jpg');
      | imagesc(bg);
      | set(ha,'handlevisibility','off', ...
      |     'visible','off')
      | uistack(ha,'top');
  Steering Wheel & Pedals : Subsystem
  Subtract2 : Sum  Inputs=+-
  Subtract3 : Sum  Inputs=+-
  Sum5 : Sum  Inputs=|++
  Sum6 : Sum  Inputs=|++
  Switch{,1..3,7,10..11} (7 alike) : Switch  Criteria=u2 > Threshold
  TIS_1_StandardCoh_Demux : Subsystem  TreatAsAtomicUnit=on  mask(PreScan Demux Block: TIS){MAXMESSAGES=1}
      mask prompts: MAXMESSAGES "Number of Objects"
      mask Help: eval('openHelp(441)')
      mask Display:
      | port_label('input',1,'TIS')
      | port_label('output',1,'Beam ID [-]')
      | port_label('output',2,'Range [m]')
      | port_label('output',3,'DopplerVelocity [m/s]')
      | port_label('output',4,'{\theta} [deg]','texmode','on')
      | port_label('output',5,'{\phi} [deg]','texmode','on')
      | port_label('output',6,'Target ID [-]','texmode','on')
      | port_label('output',7,'TIS Data','texmode','on')
  Terminator{,1..16} (17 alike) : Terminator
  Terminator_1 : Terminator
  Terminator_2 : Terminator
  Trajectories : Subsystem  Tag=Trajectories  mask(PreScan Source Block: Trajectories){}
      mask help:
      | The Trajectory block contains the trajectories defined in the PreScan Experiment Editor. The output of the trajectory block is the (vehicle) State.
      |
      | For more information, please click Help.
      settings: DeleteFcn=PreScanBlockDeleteFcn;
      mask Help: eval('openHelp(312)')
      mask Display: image(imread('Trajectory.png'));
  Video Viewer : visionsinks/Video Viewer  inputType=Obsolete7b  imagePorts=One multidimensional signal  useColorMap=off  colormapValue=gray(256)  specRange=off  minInputVal=0  maxInputVal=255  FigPos=[436 537 409 53]  AxisZoom=on  trueSizedOnce=off  OpenAtMdlStart=on  DefaultConfigurationName=vipscopes.VideoViewerScopeCfg
  aberrant driver : Display  Commented=on
  click me 1 : ManualSwitch  Commented=on
  click me 2 : ManualSwitch
  compare setting : simulink/Logic and Bit Operations/Compare To Constant  relop===  const=1  OutDataTypeStr=boolean
  compare setting1 : simulink/Logic and Bit Operations/Compare To Constant  relop=>  const=0  OutDataTypeStr=boolean
  current state is AUTO : simulink/Logic and Bit Operations/Compare To Constant  relop===  const=1  OutDataTypeStr=boolean
  current state is MANUAL : simulink/Logic and Bit Operations/Compare To Constant  relop===  const=0  OutDataTypeStr=boolean
  data logging : Subsystem
  default : Constant  Value=0
  eyetracker : Display
  h0 (meters) 1 : Constant
  hv (secs)1 : Constant  Value=1.6
  kmh1 : Gain  Gain=3.6
  kmh2 : Gain  Commented=through  Gain=3.6
  mph2 : Gain  Commented=through  Gain=.621371
  "my zero " : Constant  Value=0
  no desired  Decel1 : Constant  Value=0
  pos : Constant  Tag=pos  Value=[-399.91707801225488 254.16247682781102 339.99999999999989]
  setting : Constant
  setting1 : Constant  Value=0
  steering_ratio : Constant  Tag=steering_ratio  Value=20
  susp_front : Constant  Tag=susp_front  Value=72653
  susp_rear : Constant  Tag=susp_rear  Value=121449
  use ABERRANCE detection or  click in RT : ManualSwitch
  use COLLISION  detection or click in RT : ManualSwitch
  use COURSE  detection or click in RT1 : ManualSwitch
  STATE_Audi_A8_1 : Outport  Tag=StateOutport
  tag scope: ManualBrake=global, ManualSteer=global, On_or_Off_Road=global, Veh_X_Pos=global, Veh_Y_Pos=global, automStatus=global, cou_conf=global, speed=global
  wires:
  SELF_Demux2/10(velocity [m/s]) -> kmh2/1, Subtract2/2, PathFollower_Preview_1/6(velocity [m/s])
  kmh2/1 -> mph2/1, KMH1/1
  mph2/1 -> MPH1/1
  SELF_Demux2/1(x [m]) -> [Veh_X_Pos], SELF2PathFollowerMux1/1
  SELF_Demux2/2(y [m]) -> [Veh_Y_Pos], SELF2PathFollowerMux1/2
  SELF_Demux2/6(rotz [deg]) -> SELF2PathFollowerMux1/3
  Automation on 1/1 -> click me 2/1
  Autiomation off 0/1 -> click me 2/2
  Dynamics_Simple/2(Vx [m s-1]) -> Terminator5/1
  Switch1/1 -> Demux2/1
  Mux3/1 -> Switch1/1
  Course Conflict yes1/1 -> Double Click  to set COURSE  conflict?/1
  Course Conflict no0/1 -> Double Click  to set COURSE  conflict?/2
  Collision Conflict yes1/1 -> Double Click  to set COLLISION  conflict?/1
  Collision Conflict no0/1 -> Double Click  to set COLLISION  conflict?/2
  Double Click  to set COURSE  conflict?/1 -> use COURSE  detection or click in RT1/2
  Double Click  to set COLLISION  conflict?/1 -> use COLLISION  detection or click in RT/2
  TIS_1_StandardCoh_Demux/2(Out2) -> Subtract3/1
  Subtract2/1 -> Kv1/1
  Kp 1/1 -> Sum5/1
  Kv1/1 -> Sum5/2
  Subtract3/1 -> Kp 1/1
  hv (secs)1/1 -> Product1/1
  Product1/1 -> Sum6/2
  h0 (meters) 1/1 -> Sum6/1
  Sum6/1 -> Subtract3/2
  Compare To Zero1/1 -> Switch7/2
  no desired  Decel1/1 -> Switch7/3
  Switch7/1 -> Gain6/1
  Switch10/1 -> Dynamics_Simple/3(Brake)
  Compare To Constant6/1 -> Logical Operator9/1, Collision Conflict Detection1/1(In1), Logical Operator10/1
  Sum5/1 -> Compare To Zero1/1, Switch7/1
  Gain6/1 -> Switch10/1, Collision Conflict Detection1/2(In2)
  Switch11/1 -> Dynamics_Simple/2(Throttle)
  Gain9/1 -> Switch11/1
  Logical Operator9/1 -> Switch10/2
  Logical Operator10/1 -> Switch11/2
  Ground1/1 -> Dynamics_Simple/5(AutoManual_OnOff)
  Double Click  to set DRIVER  Abberance?/1 -> use ABERRANCE detection or  click in RT/2
  Collision Conflict Detection1/1(Out3) -> use COLLISION  detection or click in RT/1
  SELF_Demux2/7(GPS lat [deg]) -> Terminator12/1
  SELF_Demux2/8(GPS long [deg]) -> Terminator13/1
  SELF_Demux2/9(GPS alt [m]) -> Terminator14/1
  Image From File/1 -> Switch/3
  Image From File1/1 -> Switch/1
  Switch/1 -> Video Viewer/1
  SELF_Audi_A8_1/1 -> SELF_Demux2/1(SELF)
  Compare To Constant/1 -> Logical Operator1/2
  Compare To Constant1/1 -> Logical Operator1/1
  Demux2/2 -> Switch11/3, Gain9/1
  Demux2/3 -> Switch10/3
  Driver Aberrance yes1/1 -> Double Click  to set DRIVER  Abberance?/1
  Driver Aberrance no0/1 -> Double Click  to set DRIVER  Abberance?/2
  Switch2/1 -> Logical Operator10/2, Logical Operator9/2, current state is AUTO/1, [automStatus], current state is MANUAL/1, Switch/2, Switch1/2
  Logical Operator/1 -> Logical Operator4/1
  use ABERRANCE detection or  click in RT/1 -> Logical Operator/2
  use COLLISION  detection or click in RT/1 -> Logical Operator2/2
  Logical Operator2/1 -> Logical Operator/1
  Logical Operator1/1 -> [cou_conf], Course Conflict Detection/1(In1)
  Course Conflict Detection/1(Out3) -> use COURSE  detection or click in RT1/1
  use COURSE  detection or click in RT1/1 -> Logical Operator2/1
  Demux2/1 -> Dynamics_Simple/1(DeltaSteer_[deg])
  SELF_Demux2/12(yaw rate [deg/s]) -> PathFollower_Preview_1/9(Yaw rate [deg/s])
  Dynamics_Simple/3(Perf_Params) -> Bus Selector/1
  PathFollower_Preview_1/4(v0 [m/s]) -> Dynamics_Simple/4(Initial_Vx_[ms-1])
  PathFollower_Preview_1/5(Auto_GearShift) -> Dynamics_Simple/6(Auto_GearShift)
  PathFollower_Preview_1/1(delta_steerwheel [deg]) -> Mux3/1
  PathFollower_Preview_1/3(brake pressure [bar]) -> Mux3/3
  SELF2PathFollowerMux1/1 -> PathFollower_Preview_1/3(position x,y,Y [m,m,deg])
  pos/1 -> PathFollower_Preview_1/1(TrajOffset x,y,Y [m,m,deg])
  InitialVelocity/1 -> PathFollower_Preview_1/4(Initial Velocity [m/s])
  susp_front/1 -> PathFollower_Preview_1/10(CorneringStiffness_Tyres_Front [N/rad])
  susp_rear/1 -> PathFollower_Preview_1/11(CorneringStiffness_Tyres_Rear [N/rad])
  steering_ratio/1 -> PathFollower_Preview_1/12(steering_ratio[-])
  TIS_1/1 -> TIS_1_StandardCoh_Demux/1(TIS)
  Dynamics_Simple/1(State) -> STATE_Audi_A8_1/1
  Ground2/1 -> Dynamics_Simple/7(Manual_GearShift)
  SELF_Demux2/3(z [m]) -> Terminator9/1
  SELF_Demux2/4(rotx [deg]) -> Terminator10/1
  SELF_Demux2/5(roty [deg]) -> Terminator11/1
  SELF_Demux2/11(heading [deg]) -> Terminator15/1
  Bus Selector/1 -> PathFollower_Preview_1/7(vx [m/s]), kmh1/1, Speedometer/1("Speed, m/s")  "<vx_[ms-1]>"
  Bus Selector/2 -> PathFollower_Preview_1/8(vy [m/s])  "<vy_[ms-1]>"
  Mux1/1 -> Switch1/3
  PathFollower_Preview_1/6(Actor/Traj_distance [m]) -> Terminator6/1
  PathFollower_Preview_1/7(Actor/Traj_angle [deg]) -> Terminator7/1
  Eye tracking/1(output) -> use ABERRANCE detection or  click in RT/1, aberrant driver/1
  PathFollower_Preview_1/2(throttle [%]) -> Scope1/1, Switch3/3, compare setting1/1
  Steering Wheel & Pedals/1(SWA (deg)) -> Abs/1, [ManualSteer], Mux1/1
  Steering Wheel & Pedals/2(throttle (%)) -> Mux1/2
  Steering Wheel & Pedals/3(brake (bar)) -> Mux1/3, [ManualBrake]
  Eye tracking/2(message) -> eyetracker/1
  Compare To Constant2/1 -> Logical Operator3/2
  Compare To Constant3/1 -> Logical Operator3/1
  Radar_LeftBumper_Demux/2(Out1) -> Compare To Constant2/1
  Radar_RightBumper_Demux/2(Out1) -> Compare To Constant3/1
  Logical Operator3/1 -> [On_or_Off_Road]
  Radar_LeftBumper_Demux/1(activebeamID) -> Terminator4/1
  MedRdRadarRAhead_Demux/2(Out1) -> Compare To Constant/1
  MedRdRadarLAhead_Demux/2(Out1) -> Compare To Constant1/1
  Trajectories/1(State) -> Calculate Desired Velocity Automatic System Using Pythagoras2/1(State)
  Radar_RightBumper_Demux/1(activebeamID) -> Terminator3/1
  TIS_1_StandardCoh_Demux/4(Out4) -> Compare To Constant6/1
  TIS_1_StandardCoh_Demux/1(Out1) -> Terminator/1
  TIS_1_StandardCoh_Demux/3(Out3) -> Subtract2/1
  click me 2/1 -> Switch2/3
  current state is AUTO/1 -> Terminator1/1
  current state is MANUAL/1 -> Terminator2/1
  Steering Wheel & Pedals/4(buttonPress) -> Terminator8/1, Sample and Hold/Trigger
  Steering Wheel & Pedals/5(handlePull) -> Terminator16/1
  Logical Operator4/1 -> Switch2/1
  Automation on 2/1 -> Sample and Hold/1
  Automation off 3/1 -> Sample and Hold1/1
  kmh1/1 -> Display/1, [speed]
  Calculate Desired Velocity Automatic System Using Pythagoras2/1(Desired Velocity) -> PathFollower_Preview_1/5(Desired Velocity [m/s]), Scope/1
  Compare To Constant4/1 -> Sample and Hold1/Trigger
  Abs/1 -> Compare To Constant4/1
  "my zero "/1 -> Logical Operator4/2
  setting/1 -> compare setting/1, Switch2/2
  compare setting/1 -> Logical Operator5/2
  compare setting1/1 -> Logical Operator5/1
  setting1/1 -> Switch3/1
  Logical Operator5/1 -> Switch3/2
  Switch3/1 -> Mux3/2
  Radar_RightBumper/1 -> Radar_RightBumper_Demux/1(Radar)
  Radar_RightBumper_BeamData/1 -> Radar_RightBumper_Demux/2(RadarBeams)
  Radar_LeftBumper/1 -> Radar_LeftBumper_Demux/1(Radar)
  Radar_LeftBumper_BeamData/1 -> Radar_LeftBumper_Demux/2(RadarBeams)
  MedRdRadarLAhead/1 -> MedRdRadarLAhead_Demux/1(Radar)
  MedRdRadarLAhead_BeamData/1 -> MedRdRadarLAhead_Demux/2(RadarBeams)
  MedRdRadarRAhead/1 -> MedRdRadarRAhead_Demux/1(Radar)
  MedRdRadarRAhead_BeamData/1 -> MedRdRadarRAhead_Demux/2(RadarBeams)
  default/1 -> CurrentEffects_HumanView_1/1
  MedRdRadarLAhead_Demux/1(activebeamID) -> Terminator_1/1
  MedRdRadarRAhead_Demux/1(activebeamID) -> Terminator_2/1
  Ground_1/1 -> PathFollower_Preview_1/2(ActorOffset_Left(+) / Right(-) [m])
  Ground_2/1 -> Product1/2

== system W6_cs/BMW_X5_1 ==
  SELF_BMW_X5_1 : Inport  Tag=SELFInport
  SELF_Demux : Subsystem  Tag=DemuxSELF  mask(PreScan Demux Block:){}
      settings: DeleteFcn=PreScanBlockDeleteFcn;
      mask Display:
      | port_label('output',1,'x [m]')
      | port_label('output',2,'y [m]')
      | port_label('output',3,'z [m]','texmode','on')
      | port_label('output',4,'Rotx [deg]','texmode','on')
      | port_label('output',5,'Roty [deg]','texmode','on')
      | port_label('output',6,'Rotz [deg]','texmode','on')
      | port_label('output',7,'GPS lat [deg]','texmode','on')
      | port_label('output',8,'GPS long [deg]','texmode','on')
      | port_label('output',9,'GPS alt [m]','texmode','on')
      | port_label('output',10,'Velocity [m/s]')
      | port_label('output',11,'Heading [deg]')
      | port_label('output',12,'Yaw rate [deg/s]')
  Terminator_{1..12} (12 alike) : Terminator
  Trajectories : Subsystem  Tag=Trajectories  mask(PreScan Source Block: Trajectories){}
      mask help:
      | The Trajectory block contains the trajectories defined in the PreScan Experiment Editor. The output of the trajectory block is the (vehicle) State.
      |
      | For more information, please click Help.
      settings: DeleteFcn=PreScanBlockDeleteFcn;
      mask Help: eval('openHelp(312)')
      mask Display: image(imread('Trajectory.png'));
  STATE_BMW_X5_1 : Outport  Tag=StateOutport
  wires:
  SELF_BMW_X5_1/1 -> SELF_Demux/1(SELF)
  Trajectories/1(State) -> STATE_BMW_X5_1/1
  SELF_Demux/1(x [m]) -> Terminator_1/1
  SELF_Demux/2(y [m]) -> Terminator_2/1
  SELF_Demux/3(z [m]) -> Terminator_3/1
  SELF_Demux/4(rotx [deg]) -> Terminator_4/1
  SELF_Demux/5(roty [deg]) -> Terminator_5/1
  SELF_Demux/6(rotz [deg]) -> Terminator_6/1
  SELF_Demux/7(GPS lat [deg]) -> Terminator_7/1
  SELF_Demux/8(GPS long [deg]) -> Terminator_8/1
  SELF_Demux/9(GPS alt [m]) -> Terminator_9/1
  SELF_Demux/10(velocity [m/s]) -> Terminator_10/1
  SELF_Demux/11(heading [deg]) -> Terminator_11/1
  SELF_Demux/12(yaw rate [deg/s]) -> Terminator_12/1

== system W6_cs/Fiat_Bravo_1 ==
  SELF_Fiat_Bravo_1 : Inport  Tag=SELFInport
  SELF_Demux : Subsystem  Tag=DemuxSELF  mask(PreScan Demux Block:){}
      settings: DeleteFcn=PreScanBlockDeleteFcn;
      mask Display:
      | port_label('output',1,'x [m]')
      | port_label('output',2,'y [m]')
      | port_label('output',3,'z [m]','texmode','on')
      | port_label('output',4,'Rotx [deg]','texmode','on')
      | port_label('output',5,'Roty [deg]','texmode','on')
      | port_label('output',6,'Rotz [deg]','texmode','on')
      | port_label('output',7,'GPS lat [deg]','texmode','on')
      | port_label('output',8,'GPS long [deg]','texmode','on')
      | port_label('output',9,'GPS alt [m]','texmode','on')
      | port_label('output',10,'Velocity [m/s]')
      | port_label('output',11,'Heading [deg]')
      | port_label('output',12,'Yaw rate [deg/s]')
  Terminator_{1..12} (12 alike) : Terminator
  Trajectories : Subsystem  Tag=Trajectories  mask(PreScan Source Block: Trajectories){}
      mask help:
      | The Trajectory block contains the trajectories defined in the PreScan Experiment Editor. The output of the trajectory block is the (vehicle) State.
      |
      | For more information, please click Help.
      settings: DeleteFcn=PreScanBlockDeleteFcn;
      mask Help: eval('openHelp(312)')
      mask Display: image(imread('Trajectory.png'));
  STATE_Fiat_Bravo_1 : Outport  Tag=StateOutport
  wires:
  SELF_Fiat_Bravo_1/1 -> SELF_Demux/1(SELF)
  Trajectories/1(State) -> STATE_Fiat_Bravo_1/1
  SELF_Demux/1(x [m]) -> Terminator_1/1
  SELF_Demux/2(y [m]) -> Terminator_2/1
  SELF_Demux/3(z [m]) -> Terminator_3/1
  SELF_Demux/4(rotx [deg]) -> Terminator_4/1
  SELF_Demux/5(roty [deg]) -> Terminator_5/1
  SELF_Demux/6(rotz [deg]) -> Terminator_6/1
  SELF_Demux/7(GPS lat [deg]) -> Terminator_7/1
  SELF_Demux/8(GPS long [deg]) -> Terminator_8/1
  SELF_Demux/9(GPS alt [m]) -> Terminator_9/1
  SELF_Demux/10(velocity [m/s]) -> Terminator_10/1
  SELF_Demux/11(heading [deg]) -> Terminator_11/1
  SELF_Demux/12(yaw rate [deg/s]) -> Terminator_12/1
